simulink model "q2"  (R2023a)
settings: Solver=VariableStepAuto  StartTime=0.0  StopTime=10  RelTol=1e-3
settings Model: Creator=phateme  LastModifiedBy=phateme

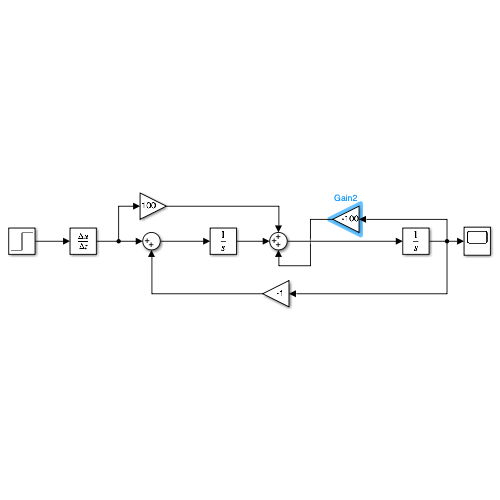
[thumbnail: Simulink's stored preview of the top-level diagram]
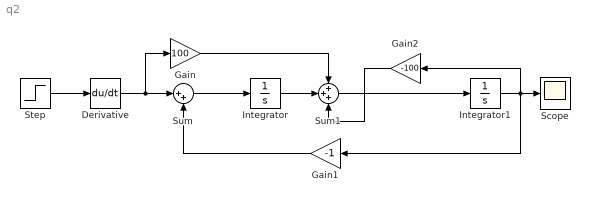
== system q2 ==
  Derivative : Derivative
  Gain : Gain  Gain=100
  Gain1 : Gain  Gain=-1
  Gain2 : Gain  Gain=-100
  Integrator : Integrator
  Integrator1 : Integrator
  Scope : Scope
  Step : Step  Time=0.001  SampleTime=0
  Sum : Sum  Inputs=|++
  Sum1 : Sum  Inputs=+++
  wires:
  Gain2/1 -> Sum1/3
  Gain1/1 -> Sum/2
  Integrator/1 -> Sum1/2
  Sum/1 -> Integrator/1
  Gain/1 -> Sum1/1
  Integrator1/1 -> Scope/1, Gain1/1, Gain2/1
  Sum1/1 -> Integrator1/1
  Derivative/1 -> Sum/1, Gain/1
  Step/1 -> Derivative/1
